simulink model "sampleModel2075"  (R2023a)
settings: Solver=VariableStepAuto  StartTime=0.0  StopTime=10.0  RelTol=1e-3
libraries: hdlsllib x3, simulink x1
settings Model: Creator=user1  LastModifiedBy=user1

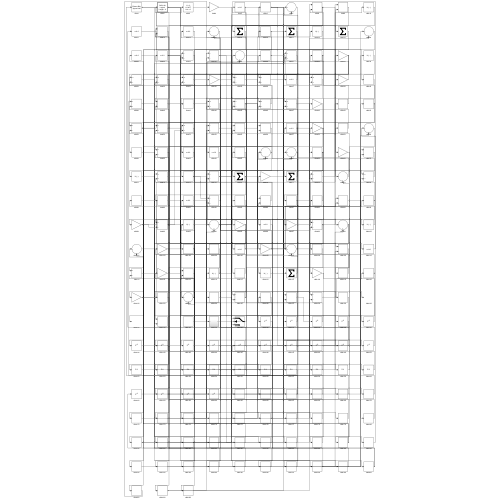
[thumbnail: Simulink's stored preview of the top-level diagram]
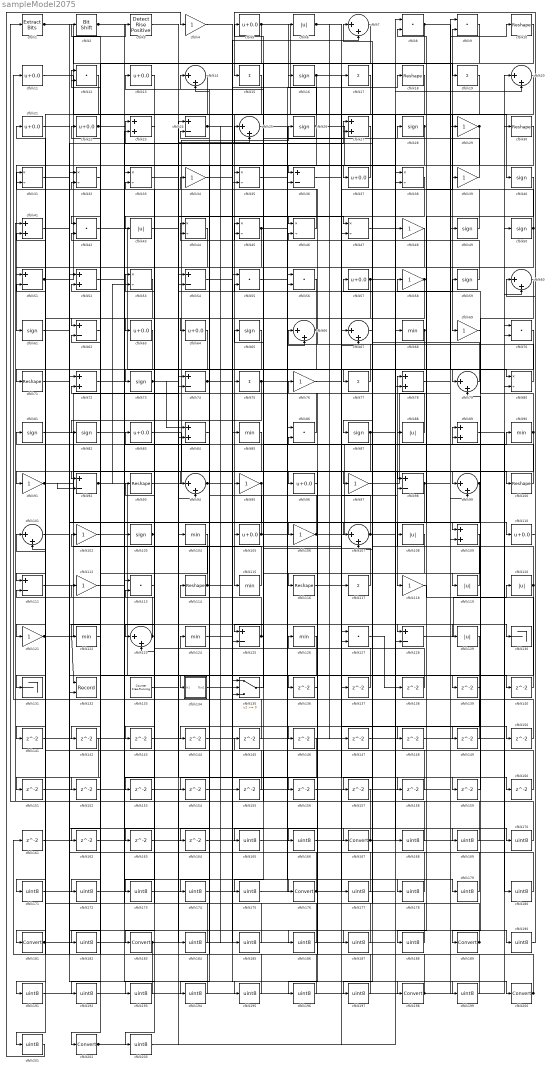
== system sampleModel2075 ==
  cfblk1 : simulink/Logic and Bit Operations/Extract Bits  bitsToExtract=Upper half  numBits=8  bitIdxRange=[0 7]  outScalingMode=Preserve fixed-point scaling
      settings: LibrarySourceBlock=|
      | hdlsllib/Logic and Bit
      | Operations/Extract Bits
  cfblk{10,18,30,71,93,100,114,116} (8 alike) : Reshape
  cfblk{7,14,20,25,60,66..67,79,94,99,101,107,123} (13 alike) : Sum  Inputs=|++
  cfblk{4,29,34,39,48,58,69,76,91,95,97,102,106,112,118,121} (16 alike) : Gain
  cfblk{16,26,28,40,49..50,59,61,65,73,81..82,87,103} (14 alike) : Signum
  cfblk{68,85,90,104,115,122,124,126} (8 alike) : MinMax
  cfblk{5,11,13,21..22,37,57,63..64,83,96,105,110} (13 alike) : Bias  Bias=0.0  SaturateOnIntegerOverflow=off
  cfblk{6,43,88,108,119..120,129} (7 alike) : Abs  SaturateOnIntegerOverflow=off
  cfblk{23,27,41,52,72,78,84,89,109} (9 alike) : Sum
  cfblk{24,36,51,54,62,74,92,98,111,125,128} (11 alike) : Sum  Inputs=+-
  cfblk{8..9,12,42,55..56,70,86,113,127} (10 alike) : DotProduct  OutDataTypeStr=Inherit: Inherit via internal rule
  cfblk{15,17,19,75,77,117} (6 alike) : Sum  Inputs=+
  cfblk130 : Terminator
  cfblk131 : Terminator
  cfblk132 : Record  FileSettingsInternal="{\"entries\":[{\"content\":{\"excelSettings\":{\"content\":{},\"type\":\"Streamout.ExcelSettings\"}},\"type\":\"Streamout.FileSettingStorage\",\"uuid\":\"\"}],\"packageUris\":[\"http:\\/\\/schema.mathworks.com\\/mf0\\/streamout_blocks\\/R2020a\"],\"version\":\"1.0\"}"  Layout=[1 1]  SignalsInternal="{\"entries\":[{\"content\":{\"signals\":[{\"content\":{\"blockPath\":[],\"dimensions\":[1],\"domain\":\"\",\"lineColor\":\"#a2142f\",\"plots\":[1],\"port\":1,\"signalID\":6512,\"signalName\":\"XY Graph:1\"},\"type\":\"RecordBlkView.Signal\",\"uuid\":\"\"},{\"content\":{\"blockPath\":[],\"dimensions\":[1],\"domain\":\"\",\"lineColor\":\"#139fff\",\"plots\":[1],\"port\":2,\"signalID\":6515,\"signalName\":\"XY Graph:2\"},\"type\":\"RecordBlkView.Signal\",\"uuid\":\"\"}]},\"type\":\"RecordBlkView.InputSignals\",\"uuid\":\"\"}],\"packageUris\":[\"http:\\/\\/schema.mathworks.com\\/mf0\\/streamout_blocks\\/R2020a\"],\"version\":\"1.0\"}"  VisualizationBindings="{\"xyplotplugin\":{\"info\":[{\"series\":[{\"bindingParametersList\":[{\"parameter\":\"X-Axis\",\"signalID\":6512,\"signalName\":\"XY Graph:1\"},{\"parameter\":\"Y-Axis\",\"signalID\":6515,\"signalName\":\"XY Graph:2\"}],\"seriesID\":4843}],\"subplotID\":1}]}}"  CompatibilityTag=XY  st=-1
  cfblk133 : hdlsllib/Sources/Counter Free-Running  NumBits=16  tsamp=-1
  cfblk134 : Subsystem
      settings: LibrarySourceBlock=|
      | hdlsllib/Ports &
      | Subsystems/Subsystem
  cfblk135 : Switch  SaturateOnIntegerOverflow=off  InputSameDT=off
  cfblk{136..164} (29 alike) : Delay  SampleTime=1
  cfblk{165..166,168..175,177..180,182,184..188,190..197,199,201,203} (31 alike) : DataTypeConversion  OutDataTypeStr=uint8  SaturateOnIntegerOverflow=off  RndMeth=Floor
  cfblk{167,176,181,183,189,198,200,202} (8 alike) : DataTypeConversion  SaturateOnIntegerOverflow=off  RndMeth=Floor
  cfblk2 : hdlsllib/Logic and Bit Operations/Bit Shift  mode=Shift Left Logical  N=0
  cfblk3 : hdlsllib/Logic and Bit Operations/Detect Rise Positive  vinit=0  OutDataTypeStr=boolean
  cfblk{31..33,35,38,44..47,53,80} (11 alike) : Product  Inputs=*/  RndMeth=Zero  SaturateOnIntegerOverflow=on
  wires:
  cfblk93/1 -> cfblk26/1
  cfblk66/1 -> cfblk64/1, cfblk94/1
  cfblk92/1 -> cfblk134/1(In1), cfblk2/1, cfblk53/2
  cfblk99/1 -> cfblk118/1, cfblk152/1
  cfblk11/1 -> cfblk69/1
  cfblk22/1 -> cfblk37/1, cfblk107/1, cfblk139/1
  cfblk15/1 -> cfblk115/1
  cfblk64/1 -> cfblk71/1
  cfblk81/1 -> cfblk106/1
  cfblk30/1 -> cfblk61/1
  cfblk83/1 -> cfblk100/1
  cfblk51/1 -> cfblk3/1, cfblk27/2
  cfblk55/1 -> cfblk27/1
  cfblk125/1 -> cfblk114/1, cfblk45/2
  cfblk110/1 -> cfblk15/1
  cfblk129/1 -> cfblk11/1
  cfblk113/1 -> cfblk183/1
  cfblk12/1 -> cfblk131/1
  cfblk6/1 -> cfblk147/1, cfblk148/1, cfblk149/1, cfblk150/1
  cfblk79/1 -> cfblk44/1
  cfblk80/1 -> cfblk66/1
  cfblk43/1 -> cfblk46/1
  cfblk42/1 -> cfblk79/1
  cfblk73/1 -> cfblk84/1, cfblk156/1
  cfblk59/1 -> cfblk46/2
  cfblk29/1 -> cfblk36/1, cfblk153/1, cfblk154/1
  cfblk50/1 -> cfblk9/2, cfblk82/1, cfblk107/2
  cfblk9/1 -> cfblk87/1
  cfblk33/1 -> cfblk25/2
  cfblk119/1 -> cfblk78/1
  cfblk84/1 -> cfblk14/1
  cfblk46/1 -> cfblk12/1
  cfblk60/1 -> cfblk189/1
  cfblk27/1 -> cfblk75/1
  cfblk17/1 -> cfblk95/1
  cfblk82/1 -> cfblk103/1
  cfblk44/1 -> cfblk51/1
  cfblk2/1 -> cfblk105/1, cfblk19/1, cfblk158/1
  cfblk105/1 -> cfblk18/1, cfblk14/2
  cfblk68/1 -> cfblk84/2, cfblk151/1
  cfblk96/1 -> cfblk116/1
  cfblk97/1 -> cfblk29/1
  cfblk115/1 -> cfblk12/2
  cfblk13/1 -> cfblk43/1
  cfblk7/1 -> cfblk42/1
  cfblk16/1 -> cfblk123/1, cfblk128/1
  cfblk117/1 -> cfblk45/1
  cfblk77/1 -> cfblk33/2
  cfblk48/1 -> cfblk181/1
  cfblk103/1 -> cfblk123/2, cfblk163/1
  cfblk4/1 -> cfblk200/1
  cfblk10/1 -> cfblk125/1
  cfblk57/1 -> cfblk62/1, cfblk169/1
  cfblk23/1 -> cfblk63/1
  cfblk112/1 -> cfblk88/1
  cfblk72/1 -> cfblk176/1
  cfblk8/1 -> cfblk80/1, cfblk125/2, cfblk135/3
  cfblk5/1 -> cfblk40/1, cfblk35/2
  cfblk133/1 -> cfblk55/2
  cfblk120/1 -> cfblk23/1, cfblk162/1
  cfblk124/1 -> cfblk198/1
  cfblk37/1 -> cfblk35/1
  cfblk104/1 -> cfblk202/1
  cfblk39/1 -> cfblk13/1
  cfblk90/1 -> cfblk58/1, cfblk91/1
  cfblk58/1 -> cfblk108/1, cfblk122/1
  cfblk91/1 -> cfblk96/1, cfblk92/2
  cfblk74/1 -> cfblk130/1, cfblk7/2
  cfblk40/1 -> cfblk98/1
  cfblk87/1 -> cfblk20/2, cfblk166/1
  cfblk86/1 -> cfblk62/2
  cfblk116/1 -> cfblk39/1
  cfblk70/1 -> cfblk78/2
  cfblk114/1 -> cfblk90/1, cfblk102/1
  cfblk24/1 -> cfblk47/1, cfblk185/1
  cfblk95/1 -> cfblk132/2, cfblk164/1
  cfblk18/1 -> cfblk73/1
  cfblk49/1 -> cfblk28/1
  cfblk26/1 -> cfblk6/1, cfblk36/2, cfblk68/1
  cfblk28/1 -> cfblk141/1, cfblk142/1
  cfblk3/1 -> cfblk77/1
  cfblk100/1 -> cfblk5/1
  cfblk128/1 -> cfblk120/1
  cfblk106/1 -> cfblk30/1, cfblk89/2, cfblk31/2
  cfblk63/1 -> cfblk111/1
  cfblk75/1 -> cfblk92/1, cfblk178/1
  cfblk121/1 -> cfblk132/1, cfblk98/2
  cfblk1/1 -> cfblk67/1, cfblk129/1
  cfblk107/1 -> cfblk81/1, cfblk160/1
  cfblk78/1 -> cfblk10/1
  cfblk45/1 -> cfblk121/1, cfblk99/1, cfblk97/1
  cfblk123/1 -> cfblk31/1, cfblk112/1
  cfblk69/1 -> cfblk119/1
  cfblk135/1 -> cfblk65/1
  cfblk98/1 -> cfblk49/1, cfblk143/1
  cfblk102/1 -> cfblk89/1
  cfblk36/1 -> cfblk127/2
  cfblk88/1 -> cfblk53/1
  cfblk111/1 -> cfblk24/1
  cfblk94/1 -> cfblk85/1, cfblk59/1, cfblk16/1
  cfblk21/1 -> cfblk110/1
  cfblk25/1 -> cfblk109/1
  cfblk20/1 -> cfblk38/2
  cfblk41/1 -> cfblk167/1
  cfblk71/1 -> cfblk136/1
  cfblk137/1 -> cfblk25/1
  cfblk127/1 -> cfblk138/1
  cfblk138/1 -> cfblk33/1
  cfblk35/1 -> cfblk140/1
  cfblk140/1 -> cfblk8/2
  cfblk141/1 -> cfblk23/2
  cfblk143/1 -> cfblk80/2
  cfblk65/1 -> cfblk144/1
  cfblk144/1 -> cfblk38/1
  cfblk145/1 -> cfblk44/2
  cfblk108/1 -> cfblk146/1
  cfblk147/1 -> cfblk9/1
  cfblk148/1 -> cfblk70/2
  cfblk149/1 -> cfblk24/2
  cfblk150/1 -> cfblk111/2
  cfblk151/1 -> cfblk66/2
  cfblk152/1 -> cfblk109/2
  cfblk154/1 -> cfblk67/2
  cfblk155/1 -> cfblk42/2
  cfblk19/1 -> cfblk157/1
  cfblk157/1 -> cfblk1/1
  cfblk158/1 -> cfblk51/2
  cfblk76/1 -> cfblk159/1
  cfblk159/1 -> cfblk79/2
  cfblk160/1 -> cfblk7/1
  cfblk161/1 -> cfblk94/2
  cfblk162/1 -> cfblk20/1
  cfblk163/1 -> cfblk74/2
  cfblk164/1 -> cfblk17/1
  cfblk126/1 -> cfblk165/1
  cfblk165/1 -> cfblk137/1
  cfblk166/1 -> cfblk126/1
  cfblk167/1 -> cfblk145/1, cfblk135/1
  cfblk47/1 -> cfblk168/1
  cfblk168/1 -> cfblk41/1
  cfblk169/1 -> cfblk41/2
  cfblk54/1 -> cfblk170/1
  cfblk170/1 -> cfblk83/1
  cfblk14/1 -> cfblk171/1
  cfblk171/1 -> cfblk54/1
  cfblk62/1 -> cfblk172/1
  cfblk172/1 -> cfblk54/2
  cfblk56/1 -> cfblk173/1
  cfblk173/1 -> cfblk8/1
  cfblk139/1 -> cfblk174/1
  cfblk174/1 -> cfblk56/1
  cfblk109/1 -> cfblk175/1
  cfblk175/1 -> cfblk56/2
  cfblk176/1 -> cfblk47/2, cfblk22/1
  cfblk156/1 -> cfblk177/1
  cfblk177/1 -> cfblk72/1
  cfblk178/1 -> cfblk72/2
  cfblk34/1 -> cfblk179/1
  cfblk179/1 -> cfblk86/1
  cfblk89/1 -> cfblk180/1
  cfblk180/1 -> cfblk34/1
  cfblk181/1 -> cfblk155/1, cfblk117/1
  cfblk122/1 -> cfblk182/1
  cfblk182/1 -> cfblk48/1
  cfblk183/1 -> cfblk161/1, cfblk55/1
  cfblk153/1 -> cfblk184/1
  cfblk184/1 -> cfblk113/1
  cfblk185/1 -> cfblk113/2
  cfblk101/1 -> cfblk186/1
  cfblk186/1 -> cfblk93/1
  cfblk134/1(Out1) -> cfblk187/1
  cfblk187/1 -> cfblk101/1
  cfblk118/1 -> cfblk188/1
  cfblk188/1 -> cfblk101/2
  cfblk189/1 -> cfblk135/2, cfblk57/1
  cfblk61/1 -> cfblk190/1
  cfblk190/1 -> cfblk60/1
  cfblk142/1 -> cfblk191/1
  cfblk191/1 -> cfblk60/2
  cfblk32/1 -> cfblk192/1
  cfblk192/1 -> cfblk50/1
  cfblk85/1 -> cfblk193/1
  cfblk193/1 -> cfblk32/1
  cfblk146/1 -> cfblk194/1
  cfblk194/1 -> cfblk32/2
  cfblk52/1 -> cfblk195/1
  cfblk195/1 -> cfblk74/1
  cfblk136/1 -> cfblk196/1
  cfblk196/1 -> cfblk52/1
  cfblk67/1 -> cfblk197/1
  cfblk197/1 -> cfblk52/2
  cfblk198/1 -> cfblk99/2, cfblk86/2, cfblk70/1
  cfblk31/1 -> cfblk199/1
  cfblk199/1 -> cfblk124/1
  cfblk200/1 -> cfblk76/1, cfblk21/1
  cfblk53/1 -> cfblk201/1
  cfblk201/1 -> cfblk4/1
  cfblk202/1 -> cfblk128/2, cfblk127/1
  cfblk38/1 -> cfblk203/1
  cfblk203/1 -> cfblk104/1

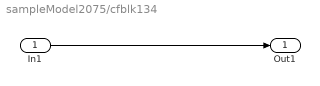
== system sampleModel2075/cfblk134 ==
  In1 : Inport
  Out1 : Outport
  wires:
  In1/1 -> Out1/1
